simulink model "cell_station_real_circuit_model_2017_214"  (R2016b)
settings: Solver=VariableStepAuto  StartTime=0.0  StopTime=120  RelTol=1e-3
undefined symbols (not defined in the file or in its folder): Acid, DiscIntNeverNeededParam, Lead, magnitude
libraries: powerlib x37, simulink x15, electricdrivelib x1, re_lib x1
settings Model: Creator=Ray Hu  LastModifiedBy=Ray Hu

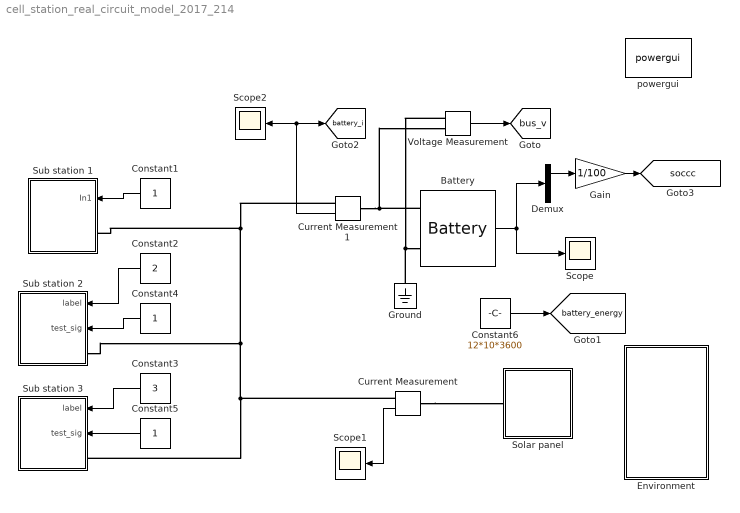
== system cell_station_real_circuit_model_2017_214 ==
  Battery : electricdrivelib/Extra Sources/Battery  BatType=Lead-Acid  ShowTempParam=off  ThermalPreset=no  NomV=12  NomQ=10  SOC=80  Batt_Tr=1  PresetModel=on  MaxQ=10.4167  MinV=9  FullV=13.0658  Dis_rate=2  R=0.012  Normal_OP=3.1028  expZone="[12.2171    0.0333333]"  current=[6.5 13 32.5]  Units=Time  Tci=20  NomT=25  T2=0  MaxQ2=2.208  FullV2=3.45  Normal_OP2=2.8  expZone2="[3.22        0.23]"  Rca=0.6  ti=1000  Dp=0
  Constant1 : Constant
  Constant2 : Constant  Value=2
  Constant3 : Constant  Value=3
  Constant4 : Constant
  Constant5 : Constant
  Constant6 : Constant  Value=12*10*3600
  Current Measurement : powerlib/Measurements/Current Measurement  PhasorSimulation=off  OutputType=Complex  PSBequivalent=0
  Current Measurement1 : powerlib/Measurements/Current Measurement  PhasorSimulation=off  OutputType=Complex  PSBequivalent=0
  Demux : Demux  Outputs=3
  Environment : Subsystem
  Gain : Gain  Gain=1/100
  Ground : powerlib/Elements/Ground  LConnTagsString=a
  Scope : Scope
  Scope1 : Scope
  Scope2 : Scope
  Solar panel : Subsystem
  Sub station 1 : Subsystem
  Sub station 2 : Subsystem
  Sub station 3 : Subsystem
  Voltage Measurement : powerlib/Measurements/Voltage Measurement  PhasorSimulation=off  OutputType=Complex  PSBequivalent=0
  powergui : powerlib/powergui  Priority=1  SimulationMode=Continuous  SolverType=Tustin/Backward Euler (TBE)  SampleTime=50e-6  frequency=60  SPID=off  DisableSnubberDevices=off  DisableRonSwitches=off  DisableVfSwitches=off  SwTol=0  DisplayEquations=off  Interpol=off  ExternalGateDelay=off  methode=off  Ts=10  FunctionMessages=off  echomessages=off  HookPort=off  EnableUseOfTLC=off  x0status=blocks  frequencyindice=0  Pbase=100e6  ErrMax=1e-4  Iterations=50  UnitsV=kV  UnitsW=MW  buscounter=0  RestoreLinks=warning  ResistiveCurrentMeasurement=off  Frange=[0:2:500]  Ylog=off  Xlog=on  ShowGrid=off  save=off  variable=ZData  structure=0  ZoomFFT=off  StartTime=0.0  cycles=1  DisplayStyle=1  fundamental=60  FreqAxis=off  MaxFrequency=1000  frequencyindicesteady=1  RmsSteady=1  display=off
  tag scope: battery_energy=global, battery_i=global, bus_v=global, soccc=global
  wires:
  Battery/1 -> Demux/1, Scope/1
  Current Measurement/1 -> Scope1/1
  Voltage Measurement/1 -> [bus_v]
  Current Measurement1/1 -> Scope2/1, [battery_i]
  Constant1/1 -> Sub station 1/1(In1)
  Constant2/1 -> Sub station 2/1(label)
  Constant3/1 -> Sub station 3/1(label)
  Demux/1 -> Gain/1
  Gain/1 -> [soccc]
  Constant4/1 -> Sub station 2/2(test_sig)
  Constant5/1 -> Sub station 3/2(test_sig)
  Constant6/1 -> [battery_energy]
  connections:
  Ground/LConn1 -- Voltage Measurement/LConn2 -- Battery/LConn2
  Current Measurement/RConn1 -- Sub station 3/LConn1 -- Sub station 2/LConn1 -- Current Measurement1/RConn1 -- Sub station 1/LConn1
  Battery/LConn1 -- Current Measurement1/LConn1 -- Voltage Measurement/LConn1
  Current Measurement/LConn1 -- Solar panel/LConn1

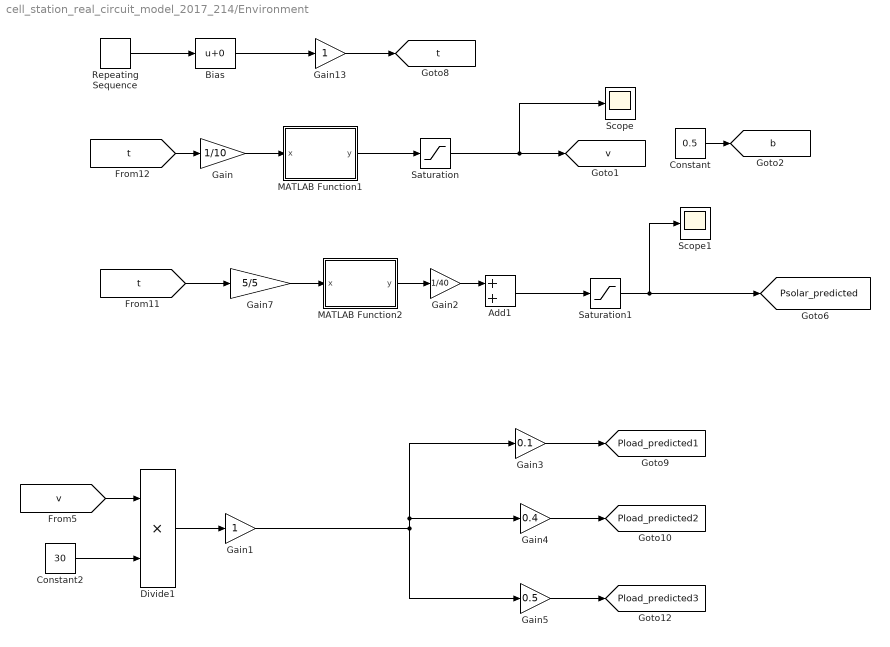
== system cell_station_real_circuit_model_2017_214/Environment ==
  Add1 : Sum
  Bias : Bias
  Constant : Constant  Value=0.5
  Constant2 : Constant  Value=30
  Divide1 : Product  Inputs=**
  Gain : Gain  Gain=1/10
  Gain1 : Gain
  Gain13 : Gain
  Gain2 : Gain  Gain=1/40
  Gain3 : Gain  Gain=0.1
  Gain4 : Gain  Gain=0.4
  Gain5 : Gain  Gain=0.5
  Gain7 : Gain  Gain=5/5
  MATLAB Function1 : MATLAB Function  TreatAsAtomicUnit=on
  MATLAB Function2 : MATLAB Function  TreatAsAtomicUnit=on
  Repeating Sequence : simulink/Sources/Repeating Sequence  rep_seq_t=[0 120]  rep_seq_y=[0 120]
  Saturation : Saturate  UpperLimit=1  LowerLimit=0
  Saturation1 : Saturate  UpperLimit=inf  LowerLimit=0
  Scope : Scope
  Scope1 : Scope
  tag scope: Pload_predicted1=global, Pload_predicted2=global, Pload_predicted3=global, Psolar_predicted=global, b=global, t=global, v=global
  wires:
  Gain7/1 -> MATLAB Function2/1(x)
  Add1/1 -> Saturation1/1
  Bias/1 -> Gain13/1
  Saturation1/1 -> Scope1/1, [Psolar_predicted]
  Gain13/1 -> [t]
  MATLAB Function2/1(y) -> Gain2/1
  Repeating Sequence/1 -> Bias/1
  [t] -> Gain7/1
  Gain2/1 -> Add1/1
  MATLAB Function1/1(y) -> Saturation/1
  Gain/1 -> MATLAB Function1/1(x)
  [t] -> Gain/1
  [v] -> Divide1/1
  Constant2/1 -> Divide1/2
  Divide1/1 -> Gain1/1
  Gain1/1 -> Gain5/1, Gain4/1, Gain3/1
  Gain3/1 -> [Pload_predicted1]
  Gain4/1 -> [Pload_predicted2]
  Gain5/1 -> [Pload_predicted3]
  Saturation/1 -> Scope/1, [v]
  Constant/1 -> [b]

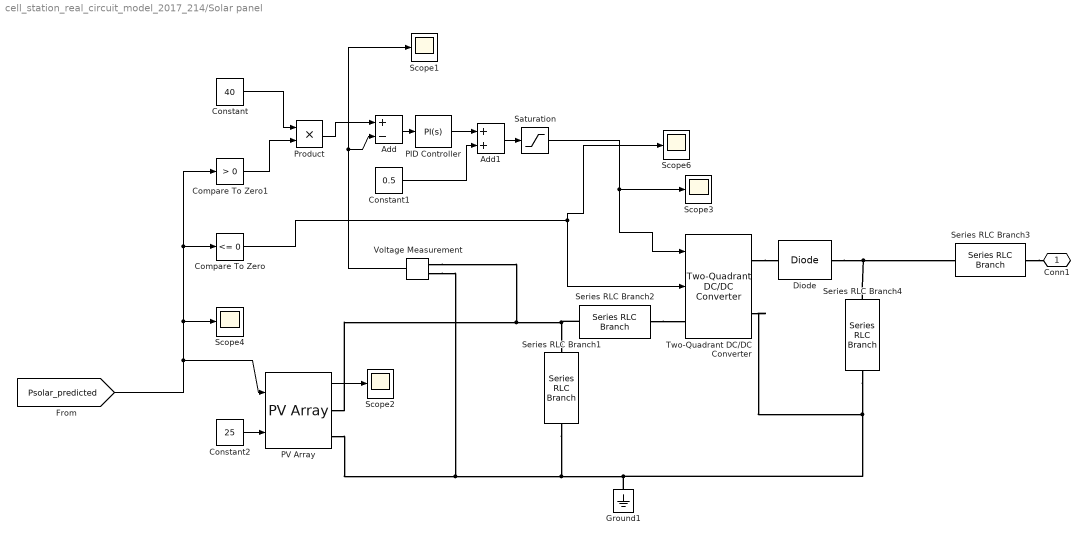
== system cell_station_real_circuit_model_2017_214/Solar panel ==
  Add : Sum  Inputs=+-
  Add1 : Sum
  Compare To Zero : simulink/Logic and Bit Operations/Compare To Zero  relop=<=  OutDataTypeStr=boolean
  Compare To Zero1 : simulink/Logic and Bit Operations/Compare To Zero  relop=>  OutDataTypeStr=boolean
  Constant : Constant  Value=40
  Constant1 : Constant  Value=0.5
  Constant2 : Constant  Value=25
  Diode : powerlib/Power Electronics/Diode  Ron=0.001  Lon=0  Vf=0.8  IC=0  UseSnubber=off  Rs=500  Cs=250e-9  Measurements=off
  Ground1 : powerlib/Elements/Ground  LConnTagsString=a
  PID Controller : simulink/Continuous/PID Controller  Controller=PI  TimeDomain=Continuous-time  SampleTime=-1  IntegratorMethod=Forward Euler  FilterMethod=Forward Euler  Form=Parallel  UseFilter=on  ControllerParametersSource=internal  P=1e-5  I=0.1  D=0  N=100  InitialConditionSource=internal  InitialConditionForIntegrator=0  InitialConditionForFilter=0  ExternalReset=none  LimitOutput=off  UpperSaturationLimit=inf  LowerSaturationLimit=-inf  LinearizeAsGain=on  AntiWindupMode=none  Kb=1  TrackingMode=off  Kt=1  PParamMin=[]  PParamMax=[]  IParamMin=[]  IParamMax=[]  DParamMin=[]  DParamMax=[]  NParamMin=[]  NParamMax=[]  KbParamMin=[]  KbParamMax=[]  KtParamMin=[]  KtParamMax=[]  POutMin=[]  POutMax=[]  IOutMin=[]  IOutMax=[]  DOutMin=[]  DOutMax=[]  NOutMin=[]  NOutMax=[]  KbOutMin=[]  KbOutMax=[]  KtOutMin=[]  KtOutMax=[]  IntegratorOutMin=[]  IntegratorOutMax=[]  FilterOutMin=[]  FilterOutMax=[]  SumOutMin=[]  SumOutMax=[]  SumI1OutMin=[]  SumI1OutMax=[]  SumI2OutMin=[]  SumI2OutMax=[]  SumI3OutMin=[]  SumI3OutMax=[]  SumDOutMin=[]  SumDOutMax=[]  SaturationOutMin=[]  SaturationOutMax=[]  IntegratorContinuousStateAttributes=''  IntegratorStateMustResolveToSignalObject=off  IntegratorRTWStateStorageClass=Auto  FilterContinuousStateAttributes=''  FilterStateMustResolveToSignalObject=off  FilterRTWStateStorageClass=Auto  DifferentiatorICPrevScaledInput=0  DifferentiatorOutMin=[]  DifferentiatorOutMax=[]
  PV Array : re_lib/Solar/PV Array  Npar=5  Nser=2  PlotType=array @ 1000 W/m2 & specified temperatures  S_vec="[ 1000  500  100 ]"  Temp_C_vec="[ 45 25  ]"  ModuleName=1Soltech 1STH-215-P  PlotWhenSelected=off  Pm=213.15  Ncell=60  Voc=36.3  Isc=7.84  Vm=29  Im=7.35  beta_Voc_pc=-0.36099  alpha_Isc_pc=0.102  beta_Voc=-0.13104  alpha_Isc=0.007997  IL=7.8649  I0=2.9259e-10  nI=0.98117  Rsh=313.3991  Rs=0.39383  BAL=off  Tc=1e-6  Tfilter=5e-5
  Product : Product
  Saturation : Saturate  UpperLimit=0.9  LowerLimit=0.1
  Scope{1..4,6} (5 alike) : Scope
  Series RLC Branch1 : powerlib/Elements/Series RLC Branch  LConnTagsString=__new0  RConnTagsString=__new0  BranchType=C  Resistance=10  Inductance=1e-3  SetiL0=off  InitialCurrent=0  Capacitance=1e-6  Setx0=on  InitialVoltage=60  Measurements=None
  Series RLC Branch2 : powerlib/Elements/Series RLC Branch  LConnTagsString=__new0  RConnTagsString=__new0  BranchType=L  Resistance=10  Inductance=1e-3  SetiL0=off  InitialCurrent=0  Capacitance=1e-6  Setx0=off  InitialVoltage=0  Measurements=None
  Series RLC Branch3 : powerlib/Elements/Series RLC Branch  LConnTagsString=__new0  RConnTagsString=__new0  BranchType=R  Resistance=0.1  Inductance=1e-6  SetiL0=off  InitialCurrent=0  Capacitance=1e-6  Setx0=off  InitialVoltage=0  Measurements=None
  Series RLC Branch4 : powerlib/Elements/Series RLC Branch  LConnTagsString=__new0  RConnTagsString=__new0  BranchType=C  Resistance=10  Inductance=1e-3  SetiL0=off  InitialCurrent=0  Capacitance=1e-6  Setx0=on  InitialVoltage=40  Measurements=None
  Two-Quadrant DC/DC Converter : powerlib/Power Electronics/Two-Quadrant DC//DC Converter  ModelType=Average model (D-controlled)  Ron=1e-3  Rs=1e6  Cs=inf  Vforward=[0,0]  Ron_Diode=1e-3  Rs_Diode=1e6  Cs_Diode=inf  Vf_Diode=1e-3  Rs_CurrentSource=inf
  Voltage Measurement : powerlib/Measurements/Voltage Measurement  PhasorSimulation=off  OutputType=Complex  PSBequivalent=0
  Conn1 : PMIOPort  Port=1  Side=Left
  wires:
  Voltage Measurement/1 -> Scope1/1, Add/2
  Add1/1 -> Saturation/1
  Constant1/1 -> Add1/2
  PID Controller/1 -> Add1/1
  Constant/1 -> Product/1
  Add/1 -> PID Controller/1
  Compare To Zero/1 -> Scope6/1, Two-Quadrant DC/DC Converter/2
  Saturation/1 -> Scope3/1, Two-Quadrant DC/DC Converter/1
  [Psolar_predicted] -> PV Array/1, Scope4/1, Compare To Zero1/1, Compare To Zero/1
  Compare To Zero1/1 -> Product/2
  Constant2/1 -> PV Array/2
  Product/1 -> Add/1
  PV Array/1 -> Scope2/1
  connections:
  Series RLC Branch3/LConn1 -- Conn1/RConn1
  Series RLC Branch1/RConn1 -- PV Array/RConn2 -- Voltage Measurement/LConn2 -- Two-Quadrant DC/DC Converter/RConn2 -- Series RLC Branch4/RConn1 -- Ground1/LConn1
  Voltage Measurement/LConn1 -- PV Array/RConn1 -- Series RLC Branch2/RConn1 -- Series RLC Branch1/LConn1
  Series RLC Branch2/LConn1 -- Two-Quadrant DC/DC Converter/LConn1
  Two-Quadrant DC/DC Converter/RConn1 -- Diode/LConn1
  Diode/RConn1 -- Series RLC Branch4/LConn1 -- Series RLC Branch3/RConn1

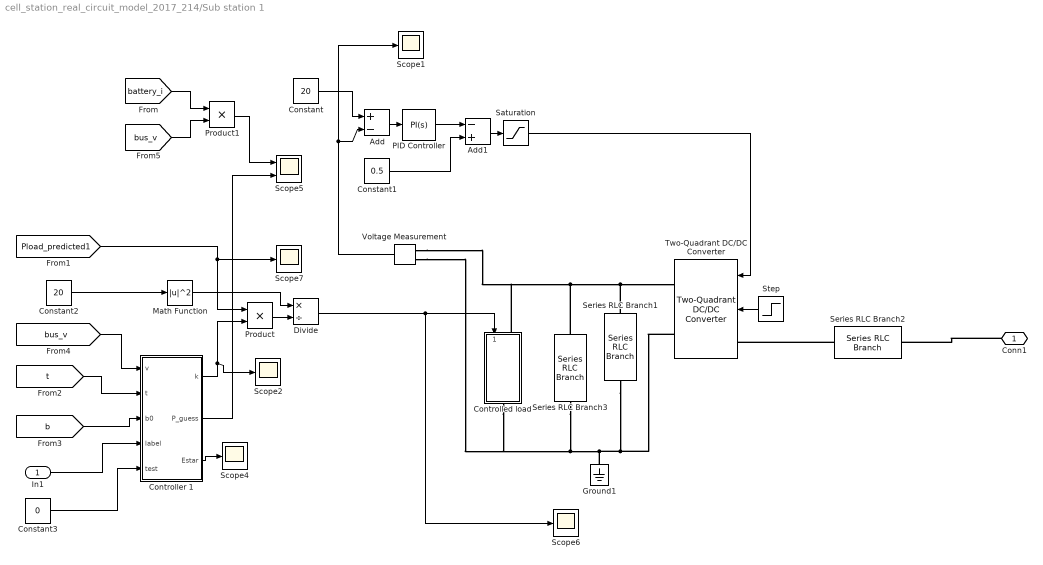
== system cell_station_real_circuit_model_2017_214/Sub station 1 ==
  In1 : Inport
  Add : Sum  Inputs=+-
  Add1 : Sum  Inputs=-+
  Constant : Constant  Value=20
  Constant1 : Constant  Value=0.5
  Constant2 : Constant  Value=20
  Constant3 : Constant  Value=0
  Controlled load : Subsystem
  Controller 1 : Subsystem
  Divide : Product  Inputs=*/
  Ground1 : powerlib/Elements/Ground  LConnTagsString=a
  Math Function : Math  Operator=magnitude^2  SaturateOnIntegerOverflow=on
  PID Controller : simulink/Continuous/PID Controller  Controller=PI  TimeDomain=Continuous-time  SampleTime=-1  IntegratorMethod=Forward Euler  FilterMethod=Forward Euler  Form=Parallel  UseFilter=on  ControllerParametersSource=internal  P=1e-5  I=0.1  D=0  N=100  InitialConditionSource=internal  InitialConditionForIntegrator=0  InitialConditionForFilter=0  ExternalReset=none  LimitOutput=off  UpperSaturationLimit=inf  LowerSaturationLimit=-inf  LinearizeAsGain=on  AntiWindupMode=none  Kb=1  TrackingMode=off  Kt=1  PParamMin=[]  PParamMax=[]  IParamMin=[]  IParamMax=[]  DParamMin=[]  DParamMax=[]  NParamMin=[]  NParamMax=[]  KbParamMin=[]  KbParamMax=[]  KtParamMin=[]  KtParamMax=[]  POutMin=[]  POutMax=[]  IOutMin=[]  IOutMax=[]  DOutMin=[]  DOutMax=[]  NOutMin=[]  NOutMax=[]  KbOutMin=[]  KbOutMax=[]  KtOutMin=[]  KtOutMax=[]  IntegratorOutMin=[]  IntegratorOutMax=[]  FilterOutMin=[]  FilterOutMax=[]  SumOutMin=[]  SumOutMax=[]  SumI1OutMin=[]  SumI1OutMax=[]  SumI2OutMin=[]  SumI2OutMax=[]  SumI3OutMin=[]  SumI3OutMax=[]  SumDOutMin=[]  SumDOutMax=[]  SaturationOutMin=[]  SaturationOutMax=[]  IntegratorContinuousStateAttributes=''  IntegratorStateMustResolveToSignalObject=off  IntegratorRTWStateStorageClass=Auto  FilterContinuousStateAttributes=''  FilterStateMustResolveToSignalObject=off  FilterRTWStateStorageClass=Auto  DifferentiatorICPrevScaledInput=0  DifferentiatorOutMin=[]  DifferentiatorOutMax=[]
  Product : Product
  Product1 : Product
  Saturation : Saturate  UpperLimit=0.9  LowerLimit=0.1
  Scope{1..2,4,6..7} (5 alike) : Scope
  Scope5 : Scope  NumInputPorts=2
  Series RLC Branch1 : powerlib/Elements/Series RLC Branch  LConnTagsString=__new0  RConnTagsString=__new0  BranchType=C  Resistance=10  Inductance=1e-3  SetiL0=off  InitialCurrent=0  Capacitance=1e-6  Setx0=on  InitialVoltage=20  Measurements=None
  Series RLC Branch2 : powerlib/Elements/Series RLC Branch  LConnTagsString=__new0  RConnTagsString=__new0  BranchType=L  Resistance=10  Inductance=1e-3  SetiL0=off  InitialCurrent=0  Capacitance=1e-6  Setx0=off  InitialVoltage=0  Measurements=None
  Series RLC Branch3 : powerlib/Elements/Series RLC Branch  LConnTagsString=__new0  RConnTagsString=__new0  BranchType=R  Resistance=100  Inductance=1e-3  SetiL0=off  InitialCurrent=0  Capacitance=1e-6  Setx0=on  InitialVoltage=60  Measurements=None
  Step : Step  Time=0  Before=1  After=0  SampleTime=0
  Two-Quadrant DC/DC Converter : powerlib/Power Electronics/Two-Quadrant DC//DC Converter  ModelType=Average model (D-controlled)  Ron=1e-3  Rs=1e6  Cs=inf  Vforward=[0,0]  Ron_Diode=1e-3  Rs_Diode=1e6  Cs_Diode=inf  Vf_Diode=1e-3  Rs_CurrentSource=inf
  Voltage Measurement : powerlib/Measurements/Voltage Measurement  PhasorSimulation=off  OutputType=Complex  PSBequivalent=0
  Conn1 : PMIOPort  Port=1  Side=Left
  wires:
  Add1/1 -> Saturation/1
  Constant1/1 -> Add1/2
  PID Controller/1 -> Add1/1
  Step/1 -> Two-Quadrant DC/DC Converter/2
  Constant/1 -> Add/1
  Saturation/1 -> Two-Quadrant DC/DC Converter/1
  Add/1 -> PID Controller/1
  Voltage Measurement/1 -> Scope1/1, Add/2
  [Pload_predicted1] -> Product/1, Scope7/1
  Controller 1/1("k ") -> Product/2, Scope2/1
  Product/1 -> Divide/2
  [t] -> Controller 1/2(t)
  [b] -> Controller 1/3(b0)
  In1/1 -> Controller 1/4(label)
  Controller 1/2(P_guess) -> Scope5/2
  Controller 1/3(Estar) -> Scope4/1
  Divide/1 -> Controlled load/1(Controllerd_R), Scope6/1
  Math Function/1 -> Divide/1
  Constant2/1 -> Math Function/1
  [bus_v] -> Controller 1/1(v)
  [battery_i] -> Product1/1
  [bus_v] -> Product1/2
  Product1/1 -> Scope5/1
  Constant3/1 -> Controller 1/5(test)
  connections:
  Conn1/RConn1 -- Series RLC Branch2/LConn1
  Series RLC Branch1/RConn1 -- Two-Quadrant DC/DC Converter/RConn2 -- Series RLC Branch3/RConn1 -- Voltage Measurement/LConn2 -- Controlled load/RConn1 -- Ground1/LConn1
  Series RLC Branch2/RConn1 -- Two-Quadrant DC/DC Converter/LConn1
  Series RLC Branch1/LConn1 -- Series RLC Branch3/LConn1 -- Voltage Measurement/LConn1 -- Controlled load/LConn1 -- Two-Quadrant DC/DC Converter/RConn1

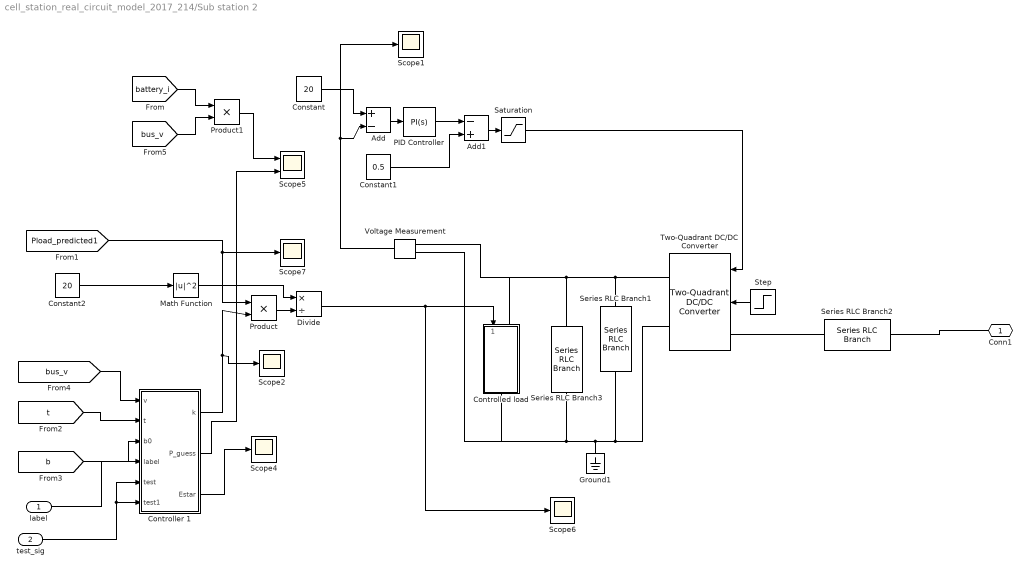
== system cell_station_real_circuit_model_2017_214/Sub station 2 ==
  label : Inport
  test_sig : Inport  Port=2
  Add : Sum  Inputs=+-
  Add1 : Sum  Inputs=-+
  Constant : Constant  Value=20
  Constant1 : Constant  Value=0.5
  Constant2 : Constant  Value=20
  Controlled load : Subsystem
  Controller 1 : Subsystem
  Divide : Product  Inputs=*/
  Ground1 : powerlib/Elements/Ground  LConnTagsString=a
  Math Function : Math  Operator=magnitude^2  SaturateOnIntegerOverflow=on
  PID Controller : simulink/Continuous/PID Controller  Controller=PI  TimeDomain=Continuous-time  SampleTime=-1  IntegratorMethod=Forward Euler  FilterMethod=Forward Euler  Form=Parallel  UseFilter=on  ControllerParametersSource=internal  P=1e-5  I=0.1  D=0  N=100  InitialConditionSource=internal  InitialConditionForIntegrator=0  InitialConditionForFilter=0  ExternalReset=none  LimitOutput=off  UpperSaturationLimit=inf  LowerSaturationLimit=-inf  LinearizeAsGain=on  AntiWindupMode=none  Kb=1  TrackingMode=off  Kt=1  PParamMin=[]  PParamMax=[]  IParamMin=[]  IParamMax=[]  DParamMin=[]  DParamMax=[]  NParamMin=[]  NParamMax=[]  KbParamMin=[]  KbParamMax=[]  KtParamMin=[]  KtParamMax=[]  POutMin=[]  POutMax=[]  IOutMin=[]  IOutMax=[]  DOutMin=[]  DOutMax=[]  NOutMin=[]  NOutMax=[]  KbOutMin=[]  KbOutMax=[]  KtOutMin=[]  KtOutMax=[]  IntegratorOutMin=[]  IntegratorOutMax=[]  FilterOutMin=[]  FilterOutMax=[]  SumOutMin=[]  SumOutMax=[]  SumI1OutMin=[]  SumI1OutMax=[]  SumI2OutMin=[]  SumI2OutMax=[]  SumI3OutMin=[]  SumI3OutMax=[]  SumDOutMin=[]  SumDOutMax=[]  SaturationOutMin=[]  SaturationOutMax=[]  IntegratorContinuousStateAttributes=''  IntegratorStateMustResolveToSignalObject=off  IntegratorRTWStateStorageClass=Auto  FilterContinuousStateAttributes=''  FilterStateMustResolveToSignalObject=off  FilterRTWStateStorageClass=Auto  DifferentiatorICPrevScaledInput=0  DifferentiatorOutMin=[]  DifferentiatorOutMax=[]
  Product : Product
  Product1 : Product
  Saturation : Saturate  UpperLimit=0.9  LowerLimit=0.1
  Scope{1..2,4,6..7} (5 alike) : Scope
  Scope5 : Scope  NumInputPorts=2
  Series RLC Branch1 : powerlib/Elements/Series RLC Branch  LConnTagsString=__new0  RConnTagsString=__new0  BranchType=C  Resistance=10  Inductance=1e-3  SetiL0=off  InitialCurrent=0  Capacitance=1e-6  Setx0=on  InitialVoltage=20  Measurements=None
  Series RLC Branch2 : powerlib/Elements/Series RLC Branch  LConnTagsString=__new0  RConnTagsString=__new0  BranchType=L  Resistance=10  Inductance=1e-3  SetiL0=off  InitialCurrent=0  Capacitance=1e-6  Setx0=off  InitialVoltage=0  Measurements=None
  Series RLC Branch3 : powerlib/Elements/Series RLC Branch  LConnTagsString=__new0  RConnTagsString=__new0  BranchType=R  Resistance=100  Inductance=1e-3  SetiL0=off  InitialCurrent=0  Capacitance=1e-6  Setx0=on  InitialVoltage=60  Measurements=None
  Step : Step  Time=0  Before=1  After=0  SampleTime=0
  Two-Quadrant DC/DC Converter : powerlib/Power Electronics/Two-Quadrant DC//DC Converter  ModelType=Average model (D-controlled)  Ron=1e-3  Rs=1e6  Cs=inf  Vforward=[0,0]  Ron_Diode=1e-3  Rs_Diode=1e6  Cs_Diode=inf  Vf_Diode=1e-3  Rs_CurrentSource=inf
  Voltage Measurement : powerlib/Measurements/Voltage Measurement  PhasorSimulation=off  OutputType=Complex  PSBequivalent=0
  Conn1 : PMIOPort  Port=1  Side=Left
  wires:
  Add1/1 -> Saturation/1
  Constant1/1 -> Add1/2
  PID Controller/1 -> Add1/1
  Step/1 -> Two-Quadrant DC/DC Converter/2
  Constant/1 -> Add/1
  Saturation/1 -> Two-Quadrant DC/DC Converter/1
  Add/1 -> PID Controller/1
  Voltage Measurement/1 -> Scope1/1, Add/2
  [Pload_predicted1] -> Product/1, Scope7/1
  Controller 1/1("k ") -> Product/2, Scope2/1
  Product/1 -> Divide/2
  [t] -> Controller 1/2(t)
  [b] -> Controller 1/3(b0)
  label/1 -> Controller 1/4(label)
  Controller 1/2(P_guess) -> Scope5/2
  Controller 1/3(Estar) -> Scope4/1
  Divide/1 -> Controlled load/1(Controllerd_R), Scope6/1
  Math Function/1 -> Divide/1
  Constant2/1 -> Math Function/1
  [bus_v] -> Controller 1/1(v)
  [battery_i] -> Product1/1
  [bus_v] -> Product1/2
  Product1/1 -> Scope5/1
  test_sig/1 -> Controller 1/6(test1), Controller 1/5(test)
  connections:
  Conn1/RConn1 -- Series RLC Branch2/LConn1
  Series RLC Branch1/RConn1 -- Two-Quadrant DC/DC Converter/RConn2 -- Series RLC Branch3/RConn1 -- Voltage Measurement/LConn2 -- Controlled load/RConn1 -- Ground1/LConn1
  Series RLC Branch2/RConn1 -- Two-Quadrant DC/DC Converter/LConn1
  Series RLC Branch1/LConn1 -- Series RLC Branch3/LConn1 -- Voltage Measurement/LConn1 -- Controlled load/LConn1 -- Two-Quadrant DC/DC Converter/RConn1

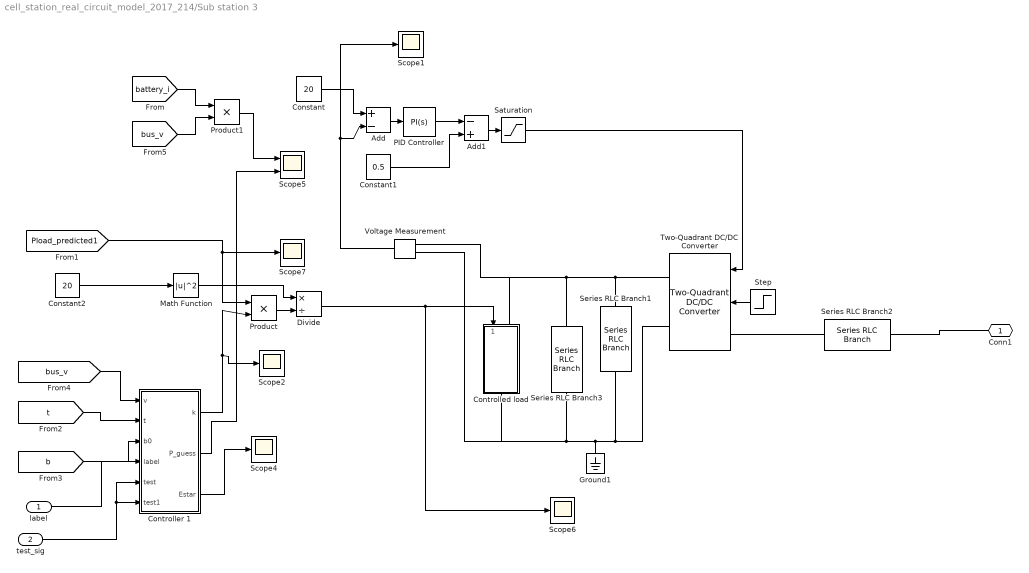
== system cell_station_real_circuit_model_2017_214/Sub station 3 ==
  label : Inport
  test_sig : Inport  Port=2
  Add : Sum  Inputs=+-
  Add1 : Sum  Inputs=-+
  Constant : Constant  Value=20
  Constant1 : Constant  Value=0.5
  Constant2 : Constant  Value=20
  Controlled load : Subsystem
  Controller 1 : Subsystem
  Divide : Product  Inputs=*/
  Ground1 : powerlib/Elements/Ground  LConnTagsString=a
  Math Function : Math  Operator=magnitude^2  SaturateOnIntegerOverflow=on
  PID Controller : simulink/Continuous/PID Controller  Controller=PI  TimeDomain=Continuous-time  SampleTime=-1  IntegratorMethod=Forward Euler  FilterMethod=Forward Euler  Form=Parallel  UseFilter=on  ControllerParametersSource=internal  P=1e-5  I=0.1  D=0  N=100  InitialConditionSource=internal  InitialConditionForIntegrator=0  InitialConditionForFilter=0  ExternalReset=none  LimitOutput=off  UpperSaturationLimit=inf  LowerSaturationLimit=-inf  LinearizeAsGain=on  AntiWindupMode=none  Kb=1  TrackingMode=off  Kt=1  PParamMin=[]  PParamMax=[]  IParamMin=[]  IParamMax=[]  DParamMin=[]  DParamMax=[]  NParamMin=[]  NParamMax=[]  KbParamMin=[]  KbParamMax=[]  KtParamMin=[]  KtParamMax=[]  POutMin=[]  POutMax=[]  IOutMin=[]  IOutMax=[]  DOutMin=[]  DOutMax=[]  NOutMin=[]  NOutMax=[]  KbOutMin=[]  KbOutMax=[]  KtOutMin=[]  KtOutMax=[]  IntegratorOutMin=[]  IntegratorOutMax=[]  FilterOutMin=[]  FilterOutMax=[]  SumOutMin=[]  SumOutMax=[]  SumI1OutMin=[]  SumI1OutMax=[]  SumI2OutMin=[]  SumI2OutMax=[]  SumI3OutMin=[]  SumI3OutMax=[]  SumDOutMin=[]  SumDOutMax=[]  SaturationOutMin=[]  SaturationOutMax=[]  IntegratorContinuousStateAttributes=''  IntegratorStateMustResolveToSignalObject=off  IntegratorRTWStateStorageClass=Auto  FilterContinuousStateAttributes=''  FilterStateMustResolveToSignalObject=off  FilterRTWStateStorageClass=Auto  DifferentiatorICPrevScaledInput=0  DifferentiatorOutMin=[]  DifferentiatorOutMax=[]
  Product : Product
  Product1 : Product
  Saturation : Saturate  UpperLimit=0.9  LowerLimit=0.1
  Scope{1..2,4,6..7} (5 alike) : Scope
  Scope5 : Scope  NumInputPorts=2
  Series RLC Branch1 : powerlib/Elements/Series RLC Branch  LConnTagsString=__new0  RConnTagsString=__new0  BranchType=C  Resistance=10  Inductance=1e-3  SetiL0=off  InitialCurrent=0  Capacitance=1e-6  Setx0=on  InitialVoltage=20  Measurements=None
  Series RLC Branch2 : powerlib/Elements/Series RLC Branch  LConnTagsString=__new0  RConnTagsString=__new0  BranchType=L  Resistance=10  Inductance=1e-3  SetiL0=off  InitialCurrent=0  Capacitance=1e-6  Setx0=off  InitialVoltage=0  Measurements=None
  Series RLC Branch3 : powerlib/Elements/Series RLC Branch  LConnTagsString=__new0  RConnTagsString=__new0  BranchType=R  Resistance=100  Inductance=1e-3  SetiL0=off  InitialCurrent=0  Capacitance=1e-6  Setx0=on  InitialVoltage=60  Measurements=None
  Step : Step  Time=0  Before=1  After=0  SampleTime=0
  Two-Quadrant DC/DC Converter : powerlib/Power Electronics/Two-Quadrant DC//DC Converter  ModelType=Average model (D-controlled)  Ron=1e-3  Rs=1e6  Cs=inf  Vforward=[0,0]  Ron_Diode=1e-3  Rs_Diode=1e6  Cs_Diode=inf  Vf_Diode=1e-3  Rs_CurrentSource=inf
  Voltage Measurement : powerlib/Measurements/Voltage Measurement  PhasorSimulation=off  OutputType=Complex  PSBequivalent=0
  Conn1 : PMIOPort  Port=1  Side=Left
  wires:
  Add1/1 -> Saturation/1
  Constant1/1 -> Add1/2
  PID Controller/1 -> Add1/1
  Step/1 -> Two-Quadrant DC/DC Converter/2
  Constant/1 -> Add/1
  Saturation/1 -> Two-Quadrant DC/DC Converter/1
  Add/1 -> PID Controller/1
  Voltage Measurement/1 -> Scope1/1, Add/2
  [Pload_predicted1] -> Product/1, Scope7/1
  Controller 1/1("k ") -> Product/2, Scope2/1
  Product/1 -> Divide/2
  [t] -> Controller 1/2(t)
  [b] -> Controller 1/3(b0)
  label/1 -> Controller 1/4(label)
  Controller 1/2(P_guess) -> Scope5/2
  Controller 1/3(Estar) -> Scope4/1
  Divide/1 -> Controlled load/1(Controllerd_R), Scope6/1
  Math Function/1 -> Divide/1
  Constant2/1 -> Math Function/1
  [bus_v] -> Controller 1/1(v)
  [battery_i] -> Product1/1
  [bus_v] -> Product1/2
  Product1/1 -> Scope5/1
  test_sig/1 -> Controller 1/6(test1), Controller 1/5(test)
  connections:
  Conn1/RConn1 -- Series RLC Branch2/LConn1
  Series RLC Branch1/RConn1 -- Two-Quadrant DC/DC Converter/RConn2 -- Series RLC Branch3/RConn1 -- Voltage Measurement/LConn2 -- Controlled load/RConn1 -- Ground1/LConn1
  Series RLC Branch2/RConn1 -- Two-Quadrant DC/DC Converter/LConn1
  Series RLC Branch1/LConn1 -- Series RLC Branch3/LConn1 -- Voltage Measurement/LConn1 -- Controlled load/LConn1 -- Two-Quadrant DC/DC Converter/RConn1

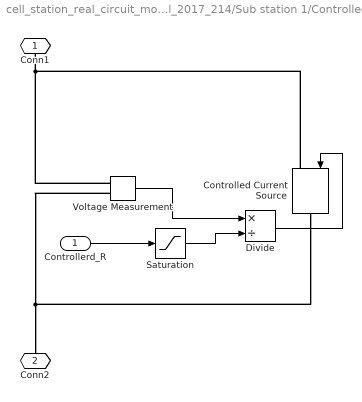
== system cell_station_real_circuit_model_2017_214/Sub station 1/Controlled load ==
  Controllerd_R : Inport
  Controlled Current Source : powerlib/Electrical Sources/Controlled Current Source  Initialize=on  Source_Type=DC  Amplitude=0  Phase=0  Frequency=0  Measurements=None
  Divide : Product  Inputs=*/
  Saturation : Saturate  UpperLimit=inf  LowerLimit=0.1
  Voltage Measurement : powerlib/Measurements/Voltage Measurement  PhasorSimulation=off  OutputType=Complex  PSBequivalent=0
  Conn1 : PMIOPort  Port=1  Side=Left
  Conn2 : PMIOPort  Port=2  Side=Right
  wires:
  Voltage Measurement/1 -> Divide/1
  Controllerd_R/1 -> Saturation/1
  Divide/1 -> Controlled Current Source/1
  Saturation/1 -> Divide/2
  connections:
  Voltage Measurement/LConn2 -- Controlled Current Source/RConn1 -- Conn2/RConn1
  Voltage Measurement/LConn1 -- Controlled Current Source/LConn1 -- Conn1/RConn1

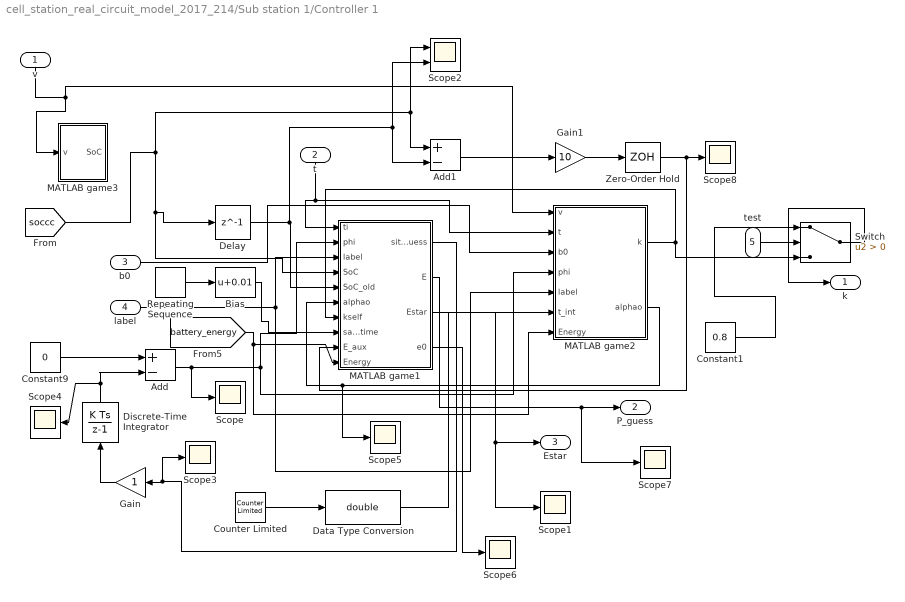
== system cell_station_real_circuit_model_2017_214/Sub station 1/Controller 1 ==
  v : Inport
  t : Inport  Port=2
  b0 : Inport  Port=3
  label : Inport  Port=4
  test : Inport  Port=5
  Add : Sum  Inputs=+-
  Add1 : Sum  Inputs=+-
  Bias : Bias  Bias=0.01
  Constant1 : Constant  Value=0.8
  Constant9 : Constant  Value=0
  Counter Limited : simulink/Sources/Counter Limited  uplimit=24  tsamp=1
  Data Type Conversion : DataTypeConversion  OutDataTypeStr=double
  Delay : Delay  DelayLength=1  InitialCondition=0  SampleTime=0.1
  Discrete-Time Integrator : DiscreteIntegrator  InitialConditionSetting=State (most efficient)  SampleTime=0.5  ICPrevOutput=DiscIntNeverNeededParam  ICPrevScaledInput=DiscIntNeverNeededParam
  Gain : Gain
  Gain1 : Gain  Gain=10
  MATLAB game1 : MATLAB Function  TreatAsAtomicUnit=on  SystemSampleTime=0.1
      settings: MinAlgLoopOccurrences=on
  MATLAB game2 : MATLAB Function  TreatAsAtomicUnit=on  SystemSampleTime=2
  MATLAB game3 : MATLAB Function  TreatAsAtomicUnit=on  SystemSampleTime=0.01
      settings: MinAlgLoopOccurrences=on
  Repeating Sequence : simulink/Sources/Repeating Sequence  rep_seq_t=[0 0.5]  rep_seq_y=[0 0.5]
  Scope{,1,3..8} (8 alike) : Scope
  Scope2 : Scope  NumInputPorts=2
  Switch : Switch  Criteria=u2 > Threshold
  Zero-Order Hold : ZeroOrderHold  SampleTime=0.1
  "k " : Outport
  P_guess : Outport  Port=2
  Estar : Outport  Port=3
  wires:
  Constant9/1 -> Add/1
  Discrete-Time Integrator/1 -> Scope4/1, Add/2
  b0/1 -> MATLAB game2/3(b0)
  Add/1 -> Scope/1, MATLAB game2/4(phi), MATLAB game1/2(phi)
  MATLAB game1/1(sitaguess) -> Scope3/1, Gain/1
  label/1 -> MATLAB game2/5(label), MATLAB game1/3(label)
  Data Type Conversion/1 -> MATLAB game2/6(t_int)
  Counter Limited/1 -> Data Type Conversion/1
  v/1 -> MATLAB game2/1(v), MATLAB game3/1(v)
  MATLAB game1/2(E) -> Scope7/1, P_guess/1
  MATLAB game2/2(alphao) -> Scope5/1, MATLAB game1/6(alphao)
  MATLAB game1/3(Estar) -> Scope1/1, Estar/1
  t/1 -> MATLAB game1/1(ti), MATLAB game2/2(t)
  MATLAB game1/4(e0) -> Scope6/1
  Delay/1 -> Add1/2, Scope2/2, MATLAB game1/5(SoC_old)
  Gain/1 -> Discrete-Time Integrator/1
  [soccc] -> MATLAB game1/4(SoC), Delay/1, Add1/1, Scope2/1
  Bias/1 -> MATLAB game1/8(sampletime)
  Repeating Sequence/1 -> Bias/1
  MATLAB game2/1(k) -> MATLAB game1/7(kself), Switch/3
  Add1/1 -> Gain1/1
  Gain1/1 -> Zero-Order Hold/1
  Zero-Order Hold/1 -> MATLAB game1/9(E_aux), Scope8/1
  Constant1/1 -> Switch/1
  Switch/1 -> "k "/1
  test/1 -> Switch/2
  [battery_energy] -> MATLAB game2/7(Energy), MATLAB game1/10(Energy)

== system cell_station_real_circuit_model_2017_214/Sub station 2/Controlled load ==
  Controllerd_R : Inport
  Controlled Current Source : powerlib/Electrical Sources/Controlled Current Source  Initialize=on  Source_Type=DC  Amplitude=0  Phase=0  Frequency=0  Measurements=None
  Divide : Product  Inputs=*/
  Saturation : Saturate  UpperLimit=inf  LowerLimit=0.1
  Voltage Measurement : powerlib/Measurements/Voltage Measurement  PhasorSimulation=off  OutputType=Complex  PSBequivalent=0
  Conn1 : PMIOPort  Port=1  Side=Left
  Conn2 : PMIOPort  Port=2  Side=Right
  wires:
  Voltage Measurement/1 -> Divide/1
  Controllerd_R/1 -> Saturation/1
  Divide/1 -> Controlled Current Source/1
  Saturation/1 -> Divide/2
  connections:
  Voltage Measurement/LConn2 -- Controlled Current Source/RConn1 -- Conn2/RConn1
  Voltage Measurement/LConn1 -- Controlled Current Source/LConn1 -- Conn1/RConn1

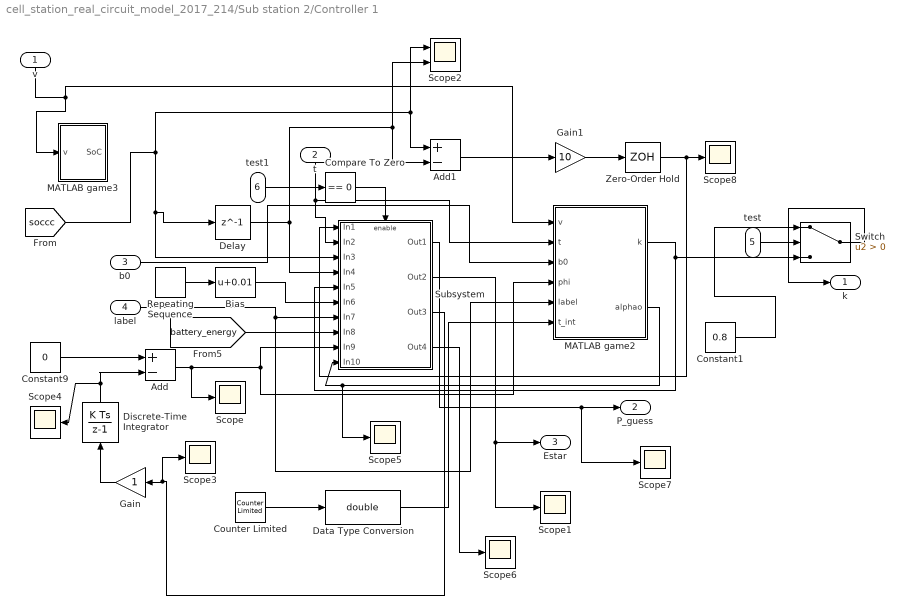
== system cell_station_real_circuit_model_2017_214/Sub station 2/Controller 1 ==
  v : Inport
  t : Inport  Port=2
  b0 : Inport  Port=3
  label : Inport  Port=4
  test : Inport  Port=5
  test1 : Inport  Port=6
  Add : Sum  Inputs=+-
  Add1 : Sum  Inputs=+-
  Bias : Bias  Bias=0.01
  Compare To Zero : simulink/Logic and Bit Operations/Compare To Zero  relop===  OutDataTypeStr=boolean
  Constant1 : Constant  Value=0.8
  Constant9 : Constant  Value=0
  Counter Limited : simulink/Sources/Counter Limited  uplimit=24  tsamp=1
  Data Type Conversion : DataTypeConversion  OutDataTypeStr=double
  Delay : Delay  DelayLength=1  InitialCondition=0  SampleTime=0.1
  Discrete-Time Integrator : DiscreteIntegrator  InitialConditionSetting=State (most efficient)  SampleTime=0.5  ICPrevOutput=DiscIntNeverNeededParam  ICPrevScaledInput=DiscIntNeverNeededParam
  Gain : Gain
  Gain1 : Gain  Gain=10
  MATLAB game2 : MATLAB Function  TreatAsAtomicUnit=on  SystemSampleTime=2
  MATLAB game3 : MATLAB Function  TreatAsAtomicUnit=on  SystemSampleTime=0.01
      settings: MinAlgLoopOccurrences=on
  Repeating Sequence : simulink/Sources/Repeating Sequence  rep_seq_t=[0 0.5]  rep_seq_y=[0 0.5]
  Scope{,1,3..8} (8 alike) : Scope
  Scope2 : Scope  NumInputPorts=2
  Subsystem : Subsystem
  Switch : Switch  Criteria=u2 > Threshold
  Zero-Order Hold : ZeroOrderHold  SampleTime=0.1
  "k " : Outport
  P_guess : Outport  Port=2
  Estar : Outport  Port=3
  wires:
  Constant9/1 -> Add/1
  Discrete-Time Integrator/1 -> Scope4/1, Add/2
  b0/1 -> MATLAB game2/3(b0)
  Add/1 -> Scope/1, Subsystem/9(In9), MATLAB game2/4(phi)
  label/1 -> Subsystem/7(In7), MATLAB game2/5(label)
  Data Type Conversion/1 -> MATLAB game2/6(t_int)
  Counter Limited/1 -> Data Type Conversion/1
  v/1 -> MATLAB game2/1(v), MATLAB game3/1(v)
  MATLAB game2/2(alphao) -> Subsystem/10(In10), Scope5/1
  t/1 -> Subsystem/2(In2), MATLAB game2/2(t)
  Delay/1 -> Subsystem/4(In4), Add1/2, Scope2/2
  Gain/1 -> Discrete-Time Integrator/1
  [soccc] -> Subsystem/3(In3), Delay/1, Add1/1, Scope2/1
  Repeating Sequence/1 -> Bias/1
  MATLAB game2/1(k) -> Subsystem/5(In5), Switch/3
  Add1/1 -> Gain1/1
  Gain1/1 -> Zero-Order Hold/1
  Zero-Order Hold/1 -> Subsystem/1(In1), Scope8/1
  Constant1/1 -> Switch/1
  Switch/1 -> "k "/1
  test/1 -> Switch/2
  Subsystem/2(Out2) -> Scope1/1, Estar/1
  Subsystem/1(Out1) -> Scope7/1, P_guess/1
  Subsystem/3(Out3) -> Scope3/1, Gain/1
  Bias/1 -> Subsystem/6(In6)
  [battery_energy] -> Subsystem/8(In8)
  Subsystem/4(Out4) -> Scope6/1
  test1/1 -> Compare To Zero/1
  Compare To Zero/1 -> Subsystem/Enable

== system cell_station_real_circuit_model_2017_214/Sub station 3/Controlled load ==
  Controllerd_R : Inport
  Controlled Current Source : powerlib/Electrical Sources/Controlled Current Source  Initialize=on  Source_Type=DC  Amplitude=0  Phase=0  Frequency=0  Measurements=None
  Divide : Product  Inputs=*/
  Saturation : Saturate  UpperLimit=inf  LowerLimit=0.1
  Voltage Measurement : powerlib/Measurements/Voltage Measurement  PhasorSimulation=off  OutputType=Complex  PSBequivalent=0
  Conn1 : PMIOPort  Port=1  Side=Left
  Conn2 : PMIOPort  Port=2  Side=Right
  wires:
  Voltage Measurement/1 -> Divide/1
  Controllerd_R/1 -> Saturation/1
  Divide/1 -> Controlled Current Source/1
  Saturation/1 -> Divide/2
  connections:
  Voltage Measurement/LConn2 -- Controlled Current Source/RConn1 -- Conn2/RConn1
  Voltage Measurement/LConn1 -- Controlled Current Source/LConn1 -- Conn1/RConn1

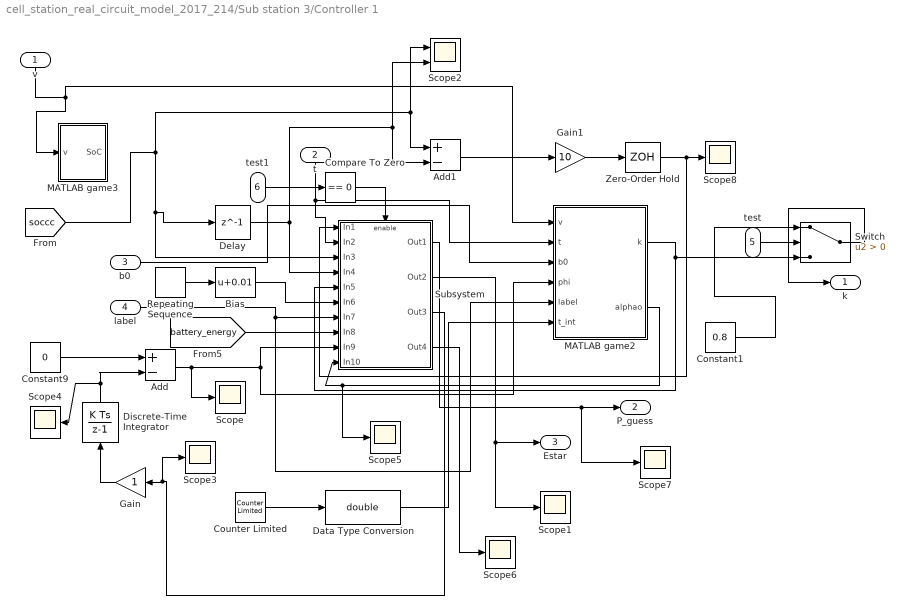
== system cell_station_real_circuit_model_2017_214/Sub station 3/Controller 1 ==
  v : Inport
  t : Inport  Port=2
  b0 : Inport  Port=3
  label : Inport  Port=4
  test : Inport  Port=5
  test1 : Inport  Port=6
  Add : Sum  Inputs=+-
  Add1 : Sum  Inputs=+-
  Bias : Bias  Bias=0.01
  Compare To Zero : simulink/Logic and Bit Operations/Compare To Zero  relop===  OutDataTypeStr=boolean
  Constant1 : Constant  Value=0.8
  Constant9 : Constant  Value=0
  Counter Limited : simulink/Sources/Counter Limited  uplimit=24  tsamp=1
  Data Type Conversion : DataTypeConversion  OutDataTypeStr=double
  Delay : Delay  DelayLength=1  InitialCondition=0  SampleTime=0.1
  Discrete-Time Integrator : DiscreteIntegrator  InitialConditionSetting=State (most efficient)  SampleTime=0.5  ICPrevOutput=DiscIntNeverNeededParam  ICPrevScaledInput=DiscIntNeverNeededParam
  Gain : Gain
  Gain1 : Gain  Gain=10
  MATLAB game2 : MATLAB Function  TreatAsAtomicUnit=on  SystemSampleTime=2
  MATLAB game3 : MATLAB Function  TreatAsAtomicUnit=on  SystemSampleTime=0.01
      settings: MinAlgLoopOccurrences=on
  Repeating Sequence : simulink/Sources/Repeating Sequence  rep_seq_t=[0 0.5]  rep_seq_y=[0 0.5]
  Scope{,1,3..8} (8 alike) : Scope
  Scope2 : Scope  NumInputPorts=2
  Subsystem : Subsystem
  Switch : Switch  Criteria=u2 > Threshold
  Zero-Order Hold : ZeroOrderHold  SampleTime=0.1
  "k " : Outport
  P_guess : Outport  Port=2
  Estar : Outport  Port=3
  wires:
  Constant9/1 -> Add/1
  Discrete-Time Integrator/1 -> Scope4/1, Add/2
  b0/1 -> MATLAB game2/3(b0)
  Add/1 -> Scope/1, Subsystem/9(In9), MATLAB game2/4(phi)
  label/1 -> Subsystem/7(In7), MATLAB game2/5(label)
  Data Type Conversion/1 -> MATLAB game2/6(t_int)
  Counter Limited/1 -> Data Type Conversion/1
  v/1 -> MATLAB game2/1(v), MATLAB game3/1(v)
  MATLAB game2/2(alphao) -> Subsystem/10(In10), Scope5/1
  t/1 -> Subsystem/2(In2), MATLAB game2/2(t)
  Delay/1 -> Subsystem/4(In4), Add1/2, Scope2/2
  Gain/1 -> Discrete-Time Integrator/1
  [soccc] -> Subsystem/3(In3), Delay/1, Add1/1, Scope2/1
  Repeating Sequence/1 -> Bias/1
  MATLAB game2/1(k) -> Subsystem/5(In5), Switch/3
  Add1/1 -> Gain1/1
  Gain1/1 -> Zero-Order Hold/1
  Zero-Order Hold/1 -> Subsystem/1(In1), Scope8/1
  Constant1/1 -> Switch/1
  Switch/1 -> "k "/1
  test/1 -> Switch/2
  Subsystem/2(Out2) -> Scope1/1, Estar/1
  Subsystem/1(Out1) -> Scope7/1, P_guess/1
  Subsystem/3(Out3) -> Scope3/1, Gain/1
  Bias/1 -> Subsystem/6(In6)
  [battery_energy] -> Subsystem/8(In8)
  Subsystem/4(Out4) -> Scope6/1
  test1/1 -> Compare To Zero/1
  Compare To Zero/1 -> Subsystem/Enable

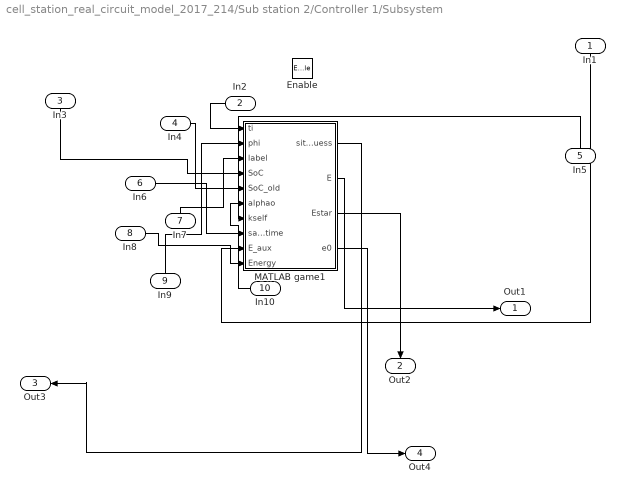
== system cell_station_real_circuit_model_2017_214/Sub station 2/Controller 1/Subsystem ==
  In1 : Inport
  In2 : Inport  Port=2
  In3 : Inport  Port=3
  In4 : Inport  Port=4
  In5 : Inport  Port=5
  In6 : Inport  Port=6
  In7 : Inport  Port=7
  In8 : Inport  Port=8
  In9 : Inport  Port=9
  In10 : Inport  Port=10
  Enable : EnablePort
  MATLAB game1 : MATLAB Function  TreatAsAtomicUnit=on  SystemSampleTime=0.1
      settings: MinAlgLoopOccurrences=on
  Out1 : Outport
  Out2 : Outport  Port=2
  Out3 : Outport  Port=3
  Out4 : Outport  Port=4
  wires:
  MATLAB game1/2(E) -> Out1/1
  MATLAB game1/1(sitaguess) -> Out3/1
  In1/1 -> MATLAB game1/9(E_aux)
  In5/1 -> MATLAB game1/7(kself)
  In2/1 -> MATLAB game1/1(ti)
  In3/1 -> MATLAB game1/4(SoC)
  In4/1 -> MATLAB game1/5(SoC_old)
  In9/1 -> MATLAB game1/2(phi)
  In10/1 -> MATLAB game1/6(alphao)
  In7/1 -> MATLAB game1/3(label)
  MATLAB game1/3(Estar) -> Out2/1
  MATLAB game1/4(e0) -> Out4/1
  In6/1 -> MATLAB game1/8(sampletime)
  In8/1 -> MATLAB game1/10(Energy)

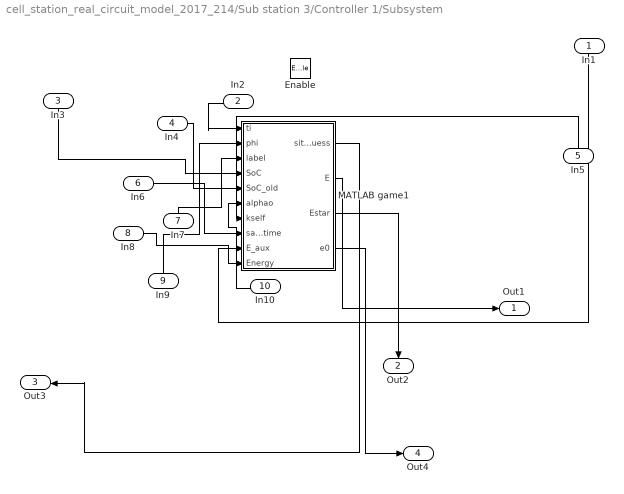
== system cell_station_real_circuit_model_2017_214/Sub station 3/Controller 1/Subsystem ==
  In1 : Inport
  In2 : Inport  Port=2
  In3 : Inport  Port=3
  In4 : Inport  Port=4
  In5 : Inport  Port=5
  In6 : Inport  Port=6
  In7 : Inport  Port=7
  In8 : Inport  Port=8
  In9 : Inport  Port=9
  In10 : Inport  Port=10
  Enable : EnablePort
  MATLAB game1 : MATLAB Function  TreatAsAtomicUnit=on  SystemSampleTime=0.1
      settings: MinAlgLoopOccurrences=on
  Out1 : Outport
  Out2 : Outport  Port=2
  Out3 : Outport  Port=3
  Out4 : Outport  Port=4
  wires:
  MATLAB game1/2(E) -> Out1/1
  MATLAB game1/1(sitaguess) -> Out3/1
  In1/1 -> MATLAB game1/9(E_aux)
  In5/1 -> MATLAB game1/7(kself)
  In2/1 -> MATLAB game1/1(ti)
  In3/1 -> MATLAB game1/4(SoC)
  In4/1 -> MATLAB game1/5(SoC_old)
  In9/1 -> MATLAB game1/2(phi)
  In10/1 -> MATLAB game1/6(alphao)
  In7/1 -> MATLAB game1/3(label)
  MATLAB game1/3(Estar) -> Out2/1
  MATLAB game1/4(e0) -> Out4/1
  In6/1 -> MATLAB game1/8(sampletime)
  In8/1 -> MATLAB game1/10(Energy)

== matlab function cell_station_real_circuit_model_2017_214/Sub station 1/Controller 1/MATLAB game3 ==
  data: v input; SoC output
function SoC = soc_detect(v)
SoC=(v-30.5)/15;

== matlab function cell_station_real_circuit_model_2017_214/Environment/MATLAB Function2 ==
  data: x input; y output
function y = fcn(x)
%#codegen
p1 =      -327.4 ;
p2 =   4.435e+04;
p3 =  -7.078e+05;
q1 =      -143.6 ;
q2 =        5928 ;
f = (p1*x^2 + p2*x + p3) / (x^2 + q1*x + q2);
y = f;

== matlab function cell_station_real_circuit_model_2017_214/Environment/MATLAB Function1 ==
  data: x input; y output
function y = fcn(x)
%#codegen

       p1 =    0.000839 ;
       p2 =       1.205  ;
       p3 =      -12.02 ;
       p4 =       34.29  ;
       q1 =      -6.495 ;
       q2 =       43.45 ;
       f = (p1*x^3 + p2*x^2 + p3*x + p4) /(x^2 + q1*x + q2);

y = f;

== matlab function cell_station_real_circuit_model_2017_214/Sub station 2/Controller 1/MATLAB game2 ==
  data: k output; v input; t input; b0 input; phi input; label input; t_int input; alphao output
function [k, alphao]  = multipleload(v,t,b0,phi,label,t_int)
wa=1-b0;
amin=1;
Energy=1*25*1000;
T=1;
batterystage=100;
n=15;
daygoal=0.8;
coder.extrinsic('linearprograming')
coder.varsize('cost1','cost2','realrow','realcolumn')
sitenumber=3;
rate=[0.1 0.4 0.5];
operation=[1,1,1];
[~, ~,alphao, k]=gamesolver_virtual_load_sinmulink(label,t_int,v,t,wa,b0,batterystage,Energy,amin,daygoal,phi,sitenumber,rate,operation);
end

== matlab function cell_station_real_circuit_model_2017_214/Sub station 2/Controller 1/MATLAB game3 ==
  data: v input; SoC output
function SoC = soc_detect(v)
SoC=(v-30.5)/15;

== matlab function cell_station_real_circuit_model_2017_214/Sub station 2/Controller 1/Subsystem/MATLAB game1 ==
  data: ti input; sitaguess output; phi input; label input; SoC input; SoC_old input; E output; alphao input; kself input; Estar output; e0 output; sampletime input; E_aux input; Energy input
function [sitaguess,E,Estar,e0] = multipleload(ti,phi,label,SoC,SoC_old,alphao,kself,sampletime,E_aux,Energy)
if SoC_old>0.1
p0=10;
t=ti/5;
rate=[0.1 0.4 0.5];

E=load2nojump(t)*rate(label)*kself+load2nojump(t)*(1-rate(label))*alphao(label)-solarnojump(t)+p0*phi;
% sampletime=0.2;
% Estar=-(SoC-SoC_old)*Energy/sampletime;
Estar=-E_aux*Energy;
if abs(Estar)>48*360
    Estar=0;
end
 e0=E-Estar;
% e0=E-po;
sitaguess=0.5e-2*(e0*p0);
else
sitaguess=0;
E=0;
Estar=0;
e0=0;
end
end
 
function Pload=load2nojump(t)
pl1 =    0.000839 ;
pl2 =       1.205  ;
pl3 =      -12.02 ;
pl4 =       34.29  ;
ql1 =      -6.495  ;
ql2 =       43.45  ;
Pload =max(0,(30* (pl1*(t).^3 + pl2*(t).^2 + pl3*(t) + pl4) ./((t).^2 + ql1*(t) + ql2))*(1+(0.2*rand-0.2*rand)*0));
end

function Psolar=solarnojump(ti)
t=ti*5;
p1 =      -327.4 ;
p2 =   4.435e+04;
p3 =  -7.078e+05;
q1 =      -143.6 ;
q2 =        5928 ;
Psolar = ((p1*t.^2 + p2*t + p3) ./ (t.^2 + q1*t + q2)+80)*(1+(0.5*rand-0.5*rand)*0)/40;
end
% 
% function [ko,koreal,alphao, kself] = gamesolver_virtual_load2(t_int,v,t,~,b0,batterystage,Energy,amin,daygoal,phi,sitenumber,rate,operation)
% alphao=zeros(1,sitenumber);
% kself=zeros(1,sitenumber);
% SoC=(v-56)*0.05+0.5;
% daygoal2=daygoal*batterystage;
% T=1;
% n=20;
% dT=T/n;
% realp=zeros(1,9);
% coder.extrinsic('linearprograming')
% coder.varsize('cost1','cost2','realrow','realcolumn')
% decide=zeros(1,sitenumber);
% P=zeros(1,batterystage*1.5);
% p=zeros(1,9);
% po=zeros(1,9);
% for ppt=1:sitenumber
%     if operation(ppt)~=0
%     opteva=zeros(9);
%     cost1=zeros(9);  
%     loadrate=rate(ppt);
% for k0=amin:1:9
%  for sigmaother0=amin:1:9
%         k=k0*0.1;
%         sigmaother=sigmaother0*0.1;       
%         [En,Sn]=pdf2_virtual_load(t,dT,loadrate,k,sigmaother,n*(24-t_int),phi(ppt));
%         if t_int~=24
%         for l=1:(batterystage*1.5)
%         P(l)=normcdf(((Energy/batterystage*(l+1)-SoC*Energy)-En*(24-t_int))/sqrt(Sn))-(normcdf(((Energy/batterystage*(l)-SoC*Energy)-En*(24-t_int))/sqrt(Sn)));
%         end
%         if (1-sum(P(1:daygoal2)))>0.5 %if there is  possibility reaching 0.8 SoC?
%             opteva(k0,sigmaother0)=b0*(sum(P(daygoal2:end)));
%             cost1(k0,sigmaother0)=((k*loadrate+sigmaother*(1-loadrate))*(1-b0)*SoC+opteva(k0,sigmaother0));
%         else  %if not stay at minimum alpha
%             cost1(k0,sigmaother0)=(1-k)/10;
%         end
%         else
%             cost1(k0,sigmaother0)=(k*loadrate+sigmaother*(1-loadrate))*(1-b0)+b0*SoC;
%         end
%  end
% end
%  [m,~]=size(cost1);
%  realrow=1:m;
% p(1:amin-1)=0;
% p(amin:9)=linearprograming(cost1(amin:9,amin:9))';
% po(1:amin-1)=0;
% po(amin:9)=linearprograming(cost1(amin:9,amin:9)')';
% linespace=0.1:0.1:0.9;
% alphao(ppt)=po*linespace';
% realn=size(realrow,2);
% for i=1:realn    
%     realp(realrow(i))=p(i);
% end
% r=rand;
% l=0;
% for i=1:9        
%     l=l+realp(i);
%     if l>r
%         break
%     end
% end
% decide(ppt)=i*0.1; 
%     end
% end
% kself=decide;
% ko=decide*rate(1:sitenumber)'/sum(rate(1:sitenumber));
% koreal=decide*rate(1:sitenumber)';
% end

== matlab function cell_station_real_circuit_model_2017_214/Sub station 3/Controller 1/Subsystem/MATLAB game1 ==
  data: ti input; sitaguess output; phi input; label input; SoC input; SoC_old input; E output; alphao input; kself input; Estar output; e0 output; sampletime input; E_aux input; Energy input
function [sitaguess,E,Estar,e0] = multipleload(ti,phi,label,SoC,SoC_old,alphao,kself,sampletime,E_aux,Energy)
if SoC_old>0.1
p0=10;
t=ti/5;
rate=[0.1 0.4 0.5];

E=load2nojump(t)*rate(label)*kself+load2nojump(t)*(1-rate(label))*alphao(label)-solarnojump(t)+p0*phi;
% sampletime=0.2;
% Estar=-(SoC-SoC_old)*Energy/sampletime;
Estar=-E_aux*Energy;
if abs(Estar)>48*360
    Estar=0;
end
 e0=E-Estar;
% e0=E-po;
sitaguess=0.5e-2*(e0*p0);
else
sitaguess=0;
E=0;
Estar=0;
e0=0;
end
end
 
function Pload=load2nojump(t)
pl1 =    0.000839 ;
pl2 =       1.205  ;
pl3 =      -12.02 ;
pl4 =       34.29  ;
ql1 =      -6.495  ;
ql2 =       43.45  ;
Pload =max(0,(30* (pl1*(t).^3 + pl2*(t).^2 + pl3*(t) + pl4) ./((t).^2 + ql1*(t) + ql2))*(1+(0.2*rand-0.2*rand)*0));
end

function Psolar=solarnojump(ti)
t=ti*5;
p1 =      -327.4 ;
p2 =   4.435e+04;
p3 =  -7.078e+05;
q1 =      -143.6 ;
q2 =        5928 ;
Psolar = ((p1*t.^2 + p2*t + p3) ./ (t.^2 + q1*t + q2)+80)*(1+(0.5*rand-0.5*rand)*0)/40;
end
% 
% function [ko,koreal,alphao, kself] = gamesolver_virtual_load2(t_int,v,t,~,b0,batterystage,Energy,amin,daygoal,phi,sitenumber,rate,operation)
% alphao=zeros(1,sitenumber);
% kself=zeros(1,sitenumber);
% SoC=(v-56)*0.05+0.5;
% daygoal2=daygoal*batterystage;
% T=1;
% n=20;
% dT=T/n;
% realp=zeros(1,9);
% coder.extrinsic('linearprograming')
% coder.varsize('cost1','cost2','realrow','realcolumn')
% decide=zeros(1,sitenumber);
% P=zeros(1,batterystage*1.5);
% p=zeros(1,9);
% po=zeros(1,9);
% for ppt=1:sitenumber
%     if operation(ppt)~=0
%     opteva=zeros(9);
%     cost1=zeros(9);  
%     loadrate=rate(ppt);
% for k0=amin:1:9
%  for sigmaother0=amin:1:9
%         k=k0*0.1;
%         sigmaother=sigmaother0*0.1;       
%         [En,Sn]=pdf2_virtual_load(t,dT,loadrate,k,sigmaother,n*(24-t_int),phi(ppt));
%         if t_int~=24
%         for l=1:(batterystage*1.5)
%         P(l)=normcdf(((Energy/batterystage*(l+1)-SoC*Energy)-En*(24-t_int))/sqrt(Sn))-(normcdf(((Energy/batterystage*(l)-SoC*Energy)-En*(24-t_int))/sqrt(Sn)));
%         end
%         if (1-sum(P(1:daygoal2)))>0.5 %if there is  possibility reaching 0.8 SoC?
%             opteva(k0,sigmaother0)=b0*(sum(P(daygoal2:end)));
%             cost1(k0,sigmaother0)=((k*loadrate+sigmaother*(1-loadrate))*(1-b0)*SoC+opteva(k0,sigmaother0));
%         else  %if not stay at minimum alpha
%             cost1(k0,sigmaother0)=(1-k)/10;
%         end
%         else
%             cost1(k0,sigmaother0)=(k*loadrate+sigmaother*(1-loadrate))*(1-b0)+b0*SoC;
%         end
%  end
% end
%  [m,~]=size(cost1);
%  realrow=1:m;
% p(1:amin-1)=0;
% p(amin:9)=linearprograming(cost1(amin:9,amin:9))';
% po(1:amin-1)=0;
% po(amin:9)=linearprograming(cost1(amin:9,amin:9)')';
% linespace=0.1:0.1:0.9;
% alphao(ppt)=po*linespace';
% realn=size(realrow,2);
% for i=1:realn    
%     realp(realrow(i))=p(i);
% end
% r=rand;
% l=0;
% for i=1:9        
%     l=l+realp(i);
%     if l>r
%         break
%     end
% end
% decide(ppt)=i*0.1; 
%     end
% end
% kself=decide;
% ko=decide*rate(1:sitenumber)'/sum(rate(1:sitenumber));
% koreal=decide*rate(1:sitenumber)';
% end

== matlab function cell_station_real_circuit_model_2017_214/Sub station 3/Controller 1/MATLAB game2 ==
  data: k output; v input; t input; b0 input; phi input; label input; t_int input; alphao output
function [k, alphao]  = multipleload(v,t,b0,phi,label,t_int)
wa=1-b0;
amin=1;
Energy=1*25*1000;
T=1;
batterystage=100;
n=15;
daygoal=0.8;
coder.extrinsic('linearprograming')
coder.varsize('cost1','cost2','realrow','realcolumn')
sitenumber=3;
rate=[0.1 0.4 0.5];
operation=[1,1,1];
[~, ~,alphao, k]=gamesolver_virtual_load_sinmulink(label,t_int,v,t,wa,b0,batterystage,Energy,amin,daygoal,phi,sitenumber,rate,operation);
end

== matlab function cell_station_real_circuit_model_2017_214/Sub station 1/Controller 1/MATLAB game1 ==
  data: ti input; sitaguess output; phi input; label input; SoC input; SoC_old input; E output; alphao input; kself input; Estar output; e0 output; sampletime input; E_aux input; Energy input
function [sitaguess,E,Estar,e0] = multipleload(ti,phi,label,SoC,SoC_old,alphao,kself,sampletime,E_aux,Energy)
if SoC_old>0.1
p0=10;
t=ti/5;
rate=[0.1 0.4 0.5];

E=load2nojump(t)*rate(label)*kself+load2nojump(t)*(1-rate(label))*alphao(label)-solarnojump(t)+p0*phi;
% sampletime=0.2;
% Estar=-(SoC-SoC_old)*Energy/sampletime;
Estar=-E_aux*Energy;
if abs(Estar)>48*360
    Estar=0;
end
 e0=E-Estar;
% e0=E-po;
sitaguess=0.5e-2*(e0*p0);
else
sitaguess=0;
E=0;
Estar=0;
e0=0;
end
end
 
function Pload=load2nojump(t)
pl1 =    0.000839 ;
pl2 =       1.205  ;
pl3 =      -12.02 ;
pl4 =       34.29  ;
ql1 =      -6.495  ;
ql2 =       43.45  ;
Pload =max(0,(30* (pl1*(t).^3 + pl2*(t).^2 + pl3*(t) + pl4) ./((t).^2 + ql1*(t) + ql2))*(1+(0.2*rand-0.2*rand)*0));
end

function Psolar=solarnojump(ti)
t=ti*5;
p1 =      -327.4 ;
p2 =   4.435e+04;
p3 =  -7.078e+05;
q1 =      -143.6 ;
q2 =        5928 ;
Psolar = ((p1*t.^2 + p2*t + p3) ./ (t.^2 + q1*t + q2)+80)*(1+(0.5*rand-0.5*rand)*0)/40;
end
% 
% function [ko,koreal,alphao, kself] = gamesolver_virtual_load2(t_int,v,t,~,b0,batterystage,Energy,amin,daygoal,phi,sitenumber,rate,operation)
% alphao=zeros(1,sitenumber);
% kself=zeros(1,sitenumber);
% SoC=(v-56)*0.05+0.5;
% daygoal2=daygoal*batterystage;
% T=1;
% n=20;
% dT=T/n;
% realp=zeros(1,9);
% coder.extrinsic('linearprograming')
% coder.varsize('cost1','cost2','realrow','realcolumn')
% decide=zeros(1,sitenumber);
% P=zeros(1,batterystage*1.5);
% p=zeros(1,9);
% po=zeros(1,9);
% for ppt=1:sitenumber
%     if operation(ppt)~=0
%     opteva=zeros(9);
%     cost1=zeros(9);  
%     loadrate=rate(ppt);
% for k0=amin:1:9
%  for sigmaother0=amin:1:9
%         k=k0*0.1;
%         sigmaother=sigmaother0*0.1;       
%         [En,Sn]=pdf2_virtual_load(t,dT,loadrate,k,sigmaother,n*(24-t_int),phi(ppt));
%         if t_int~=24
%         for l=1:(batterystage*1.5)
%         P(l)=normcdf(((Energy/batterystage*(l+1)-SoC*Energy)-En*(24-t_int))/sqrt(Sn))-(normcdf(((Energy/batterystage*(l)-SoC*Energy)-En*(24-t_int))/sqrt(Sn)));
%         end
%         if (1-sum(P(1:daygoal2)))>0.5 %if there is  possibility reaching 0.8 SoC?
%             opteva(k0,sigmaother0)=b0*(sum(P(daygoal2:end)));
%             cost1(k0,sigmaother0)=((k*loadrate+sigmaother*(1-loadrate))*(1-b0)*SoC+opteva(k0,sigmaother0));
%         else  %if not stay at minimum alpha
%             cost1(k0,sigmaother0)=(1-k)/10;
%         end
%         else
%             cost1(k0,sigmaother0)=(k*loadrate+sigmaother*(1-loadrate))*(1-b0)+b0*SoC;
%         end
%  end
% end
%  [m,~]=size(cost1);
%  realrow=1:m;
% p(1:amin-1)=0;
% p(amin:9)=linearprograming(cost1(amin:9,amin:9))';
% po(1:amin-1)=0;
% po(amin:9)=linearprograming(cost1(amin:9,amin:9)')';
% linespace=0.1:0.1:0.9;
% alphao(ppt)=po*linespace';
% realn=size(realrow,2);
% for i=1:realn    
%     realp(realrow(i))=p(i);
% end
% r=rand;
% l=0;
% for i=1:9        
%     l=l+realp(i);
%     if l>r
%         break
%     end
% end
% decide(ppt)=i*0.1; 
%     end
% end
% kself=decide;
% ko=decide*rate(1:sitenumber)'/sum(rate(1:sitenumber));
% koreal=decide*rate(1:sitenumber)';
% end

== matlab function cell_station_real_circuit_model_2017_214/Sub station 1/Controller 1/MATLAB game2 ==
  data: k output; v input; t input; b0 input; phi input; label input; t_int input; alphao output; Energy input
function [k, alphao]  = multipleload(v,t,b0,phi,label,t_int,Energy)
wa=1-b0;
amin=1;

T=1;
batterystage=100;
n=15;
daygoal=0.8;
coder.extrinsic('linearprograming')
coder.varsize('cost1','cost2','realrow','realcolumn')
sitenumber=3;
rate=[0.1 0.4 0.5];
operation=[1,1,1];
[~, ~,alphao, k]=gamesolver_virtual_load_sinmulink(label,t_int,v,t,wa,b0,batterystage,Energy,amin,daygoal,phi,sitenumber,rate,operation);
end

== matlab function cell_station_real_circuit_model_2017_214/Sub station 3/Controller 1/MATLAB game3 ==
  data: v input; SoC output
function SoC = soc_detect(v)
SoC=(v-30.5)/15;
